simulink model "VehicleModel2kmph"  (R2018a)
settings: Solver=VariableStepAuto  StartTime=0.0  StopTime=1220  RelTol=1e-3
libraries: qss_tb_library x2, simulink x2
settings Model: Creator=egp  LastModifiedBy=egp

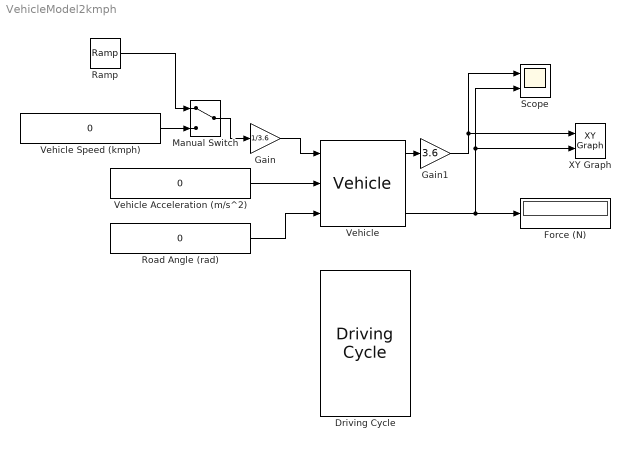
== system VehicleModel2kmph ==
  Driving Cycle : qss_tb_library/Driving Cycle/Driving Cycle  Tag=cycle  cyclename1=NEDC  stepsize=1  autostop=on
  Force (N) : Display
  Gain : Gain  Gain=1/3.6
  Gain1 : Gain  Gain=3.6
  Manual Switch : ManualSwitch
  Ramp : simulink/Sources/Ramp  slope=60/10  start=0  InitialOutput=0
  Road Angle (rad) : Constant  Value=0
  Scope : Scope  NumInputPorts=2
  Vehicle : qss_tb_library/Vehicle/Vehicle  Tag=vehicle  m_f=1750  A_f=2.88  cw=0.5  mu=0.01  k_inertia=5
  Vehicle Acceleration (m/s^2) : Constant  Value=0
  Vehicle Speed (kmph) : Constant  Value=0
  XY Graph : simulink/Sinks/XY Graph  xmin=0  xmax=60  ymin=0  ymax=500  st=-1
  wires:
  Road Angle (rad)/1 -> Vehicle/3
  Vehicle Acceleration (m/s^2)/1 -> Vehicle/2
  Vehicle/3 -> XY Graph/2, Scope/2, Force (N)/1
  Vehicle Speed (kmph)/1 -> Manual Switch/2
  Ramp/1 -> Manual Switch/1
  Manual Switch/1 -> Gain/1
  Gain/1 -> Vehicle/1
  Vehicle/1 -> Gain1/1
  Gain1/1 -> XY Graph/1, Scope/1
